simulink model "dfeq"  (Simulink 7.6)
settings: Solver=ode45  StartTime=0.0  StopTime=10.0  RelTol=1e-3
libraries: fuzblock x1
settings Model: Creator=kif  LastModifiedBy=kif

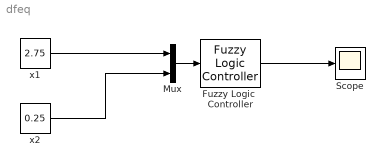
== system dfeq ==
  Fuzzy Logic  Controller : fuzblock/Fuzzy Logic  Controller  SystemSampleTime=-1  fis=takaji
  Mux : Mux  Inputs=2
  Scope : Scope
  x1 : Constant  Value=2.75
  x2 : Constant  Value=0.25
  wires:
  Mux/1 -> Fuzzy Logic  Controller/1
  x1/1 -> Mux/1
  x2/1 -> Mux/2
  Fuzzy Logic  Controller/1 -> Scope/1
